simulink model "Stepper_Model_Statespace_Controller"  (R2017a)
settings: Solver=VariableStepAuto  StartTime=0.0  StopTime=15  FixedStep=0.01  RelTol=1e-3
undefined symbols (not defined in the file): Ad, Bd, Cd, Dd, Ptheta0, T, theta0
libraries: simulink x2
settings Model: Creator=Patrick  LastModifiedBy=Patrick

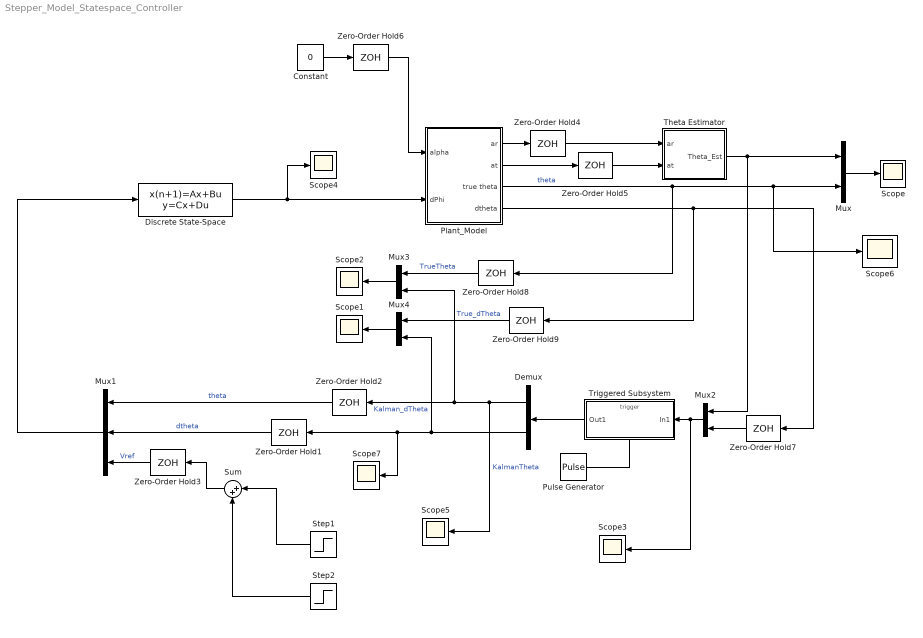
== system Stepper_Model_Statespace_Controller ==
  Constant : Constant  Value=0
  Demux : Demux  Outputs=2
  Discrete State-Space : DiscreteStateSpace  A=Ad  B=Bd  C=Cd  D=Dd  SampleTime=T
  Mux{,2..4} (4 alike) : Mux  Inputs=2
  Mux1 : Mux  Inputs=3
  Plant_Model : Subsystem
  Pulse Generator : DiscretePulseGenerator  PulseType=Time based  Period=T  PulseWidth=50
  Scope{,1..7} (8 alike) : Scope
  Step1 : Step  Time=5  After=.5  SampleTime=0
  Step2 : Step  Time=10  After=0  SampleTime=0
  Sum : Sum  Inputs=|++
  Theta Estimator : Subsystem
  Triggered Subsystem : Subsystem  TreatAsAtomicUnit=on
  Zero-Order Hold{1..9} (9 alike) : ZeroOrderHold  SampleTime=T
  wires:
  Mux/1 -> Scope/1
  Plant_Model/3(true theta) -> Scope6/1, Mux/2, Zero-Order Hold8/1  "theta"
  Mux1/1 -> Discrete State-Space/1
  Discrete State-Space/1 -> Scope4/1, Plant_Model/2(dPhi)
  Zero-Order Hold1/1 -> Mux1/2  "dtheta"
  Zero-Order Hold2/1 -> Mux1/1  "theta"
  Zero-Order Hold3/1 -> Mux1/3  "Vref"
  Plant_Model/1(ar) -> Zero-Order Hold4/1
  Zero-Order Hold4/1 -> Theta Estimator/1(ar)
  Zero-Order Hold5/1 -> Theta Estimator/2(at)
  Plant_Model/2(at) -> Zero-Order Hold5/1
  Theta Estimator/1(Theta_Est) -> Mux/1, Mux2/1
  Triggered Subsystem/1(Out1) -> Demux/1
  Mux2/1 -> Scope3/1, Triggered Subsystem/1(In1)
  Plant_Model/4(dtheta) -> Zero-Order Hold7/1, Zero-Order Hold9/1
  Mux3/1 -> Scope2/1
  Mux4/1 -> Scope1/1
  Demux/2 -> Scope7/1, Zero-Order Hold1/1, Mux4/2  "Kalman_dTheta"
  Demux/1 -> Scope5/1, Zero-Order Hold2/1, Mux3/2  "KalmanTheta"
  Pulse Generator/1 -> Triggered Subsystem/Trigger
  Zero-Order Hold7/1 -> Mux2/2
  Constant/1 -> Zero-Order Hold6/1
  Zero-Order Hold6/1 -> Plant_Model/1("alpha ")
  Zero-Order Hold8/1 -> Mux3/1  "TrueTheta"
  Zero-Order Hold9/1 -> Mux4/1  "True_dTheta"
  Sum/1 -> Zero-Order Hold3/1
  Step1/1 -> Sum/1
  Step2/1 -> Sum/2

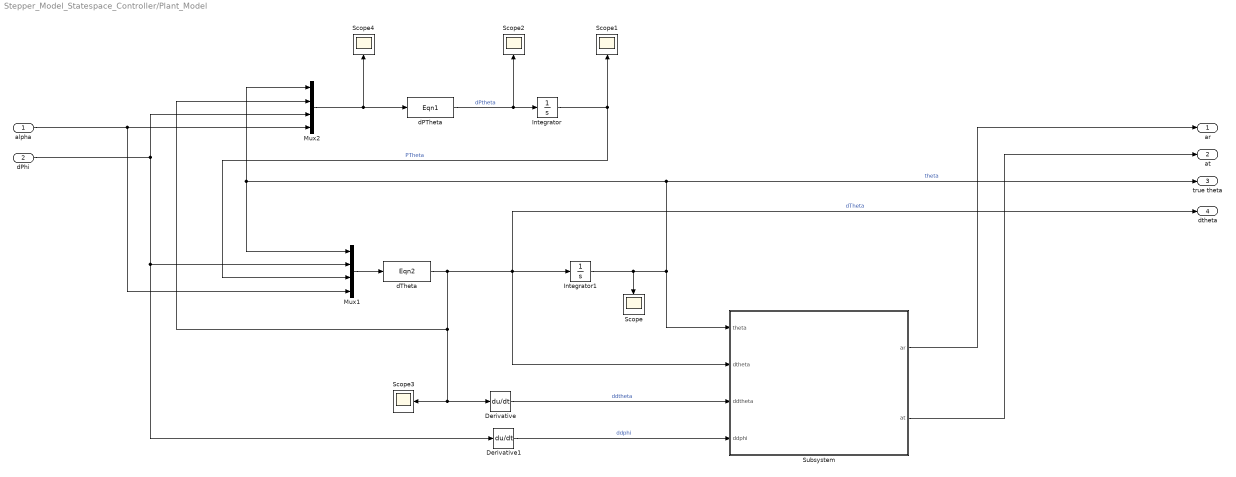
== system Stepper_Model_Statespace_Controller/Plant_Model ==
  "alpha " : Inport
  dPhi : Inport  Port=2
  Derivative : Derivative
  Derivative1 : Derivative
  Integrator : Integrator  InitialCondition=Ptheta0
  Integrator1 : Integrator  InitialCondition=theta0
  Mux1 : Mux  Inputs=[1 1 1 1]
  Mux2 : Mux  Inputs=[1 1 1 1]
  Scope{,1..4} (5 alike) : Scope
  Subsystem : Subsystem
  dPTheta : MATLABFcn  MATLABFcn=Eqn1  OutputDimensions=[1 1]  Output1D=off
  dTheta : MATLABFcn  MATLABFcn=Eqn2  OutputDimensions=[1 1]  Output1D=off
  ar : Outport  PortDimensions=[1 1]
  at : Outport  Port=2  PortDimensions=[1 1]
  true theta : Outport  Port=3  PortDimensions=[1 1]
  dtheta : Outport  Port=4  PortDimensions=[1 1]
  wires:
  Integrator/1 -> Mux1/3, Scope1/1  "PTheta"
  dPTheta/1 -> Integrator/1, Scope2/1  "dPtheta"
  dTheta/1 -> Subsystem/2(dtheta), dtheta/1, Integrator1/1, Scope3/1, Derivative/1, Mux2/2  "dTheta"
  Mux2/1 -> dPTheta/1, Scope4/1
  Mux1/1 -> dTheta/1
  Derivative/1 -> Subsystem/3(ddtheta)  "ddtheta"
  Derivative1/1 -> Subsystem/4(ddphi)  "ddphi"
  Integrator1/1 -> Subsystem/1(theta), Mux2/1, Mux1/1, true theta/1, Scope/1  "theta"
  Subsystem/2(at) -> at/1
  Subsystem/1(ar) -> ar/1
  dPhi/1 -> Derivative1/1, Mux1/2, Mux2/3
  "alpha "/1 -> Mux1/4, Mux2/4

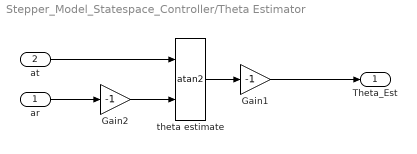
== system Stepper_Model_Statespace_Controller/Theta Estimator ==
  ar : Inport
  at : Inport  Port=2
  Gain1 : Gain  Gain=-1
  Gain2 : Gain  Gain=-1
  theta estimate : Trigonometry  Operator=atan2  OutputSignalType=real
  Theta_Est : Outport
  wires:
  ar/1 -> Gain2/1
  at/1 -> theta estimate/1
  Gain2/1 -> theta estimate/2
  theta estimate/1 -> Gain1/1
  Gain1/1 -> Theta_Est/1

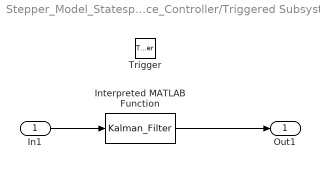
== system Stepper_Model_Statespace_Controller/Triggered Subsystem ==
  In1 : Inport
  Trigger : TriggerPort  VariantControl=Variant
  Interpreted MATLAB Function : MATLABFcn  MATLABFcn=Kalman_Filter  OutputDimensions=[2, 1]  Output1D=off
  Out1 : Outport
  wires:
  In1/1 -> Interpreted MATLAB Function/1
  Interpreted MATLAB Function/1 -> Out1/1

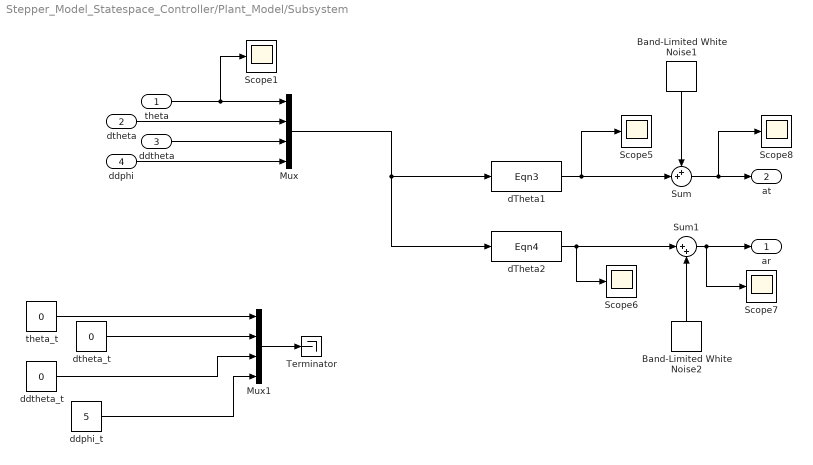
== system Stepper_Model_Statespace_Controller/Plant_Model/Subsystem ==
  theta : Inport
  dtheta : Inport  Port=2
  ddtheta : Inport  Port=3
  ddphi : Inport  Port=4
  Band-Limited White Noise1 : simulink/Sources/Band-Limited White Noise  Cov=[0.0000001]  Ts=.01  seed=[23341]
  Band-Limited White Noise2 : simulink/Sources/Band-Limited White Noise  Cov=[0.00000001]  Ts=.01  seed=[23341]
  Mux : Mux
  Mux1 : Mux
  Scope{1,5..8} (5 alike) : Scope
  Sum : Sum  Inputs=++|
  Sum1 : Sum  Inputs=|++
  Terminator : Terminator
  dTheta1 : MATLABFcn  MATLABFcn=Eqn3  OutputDimensions=[1 1]  Output1D=off
  dTheta2 : MATLABFcn  MATLABFcn=Eqn4  OutputDimensions=[1 1]  Output1D=off
  ddphi_t : Constant  Value=5
  ddtheta_t : Constant  Value=0
  dtheta_t : Constant  Value=0
  theta_t : Constant  Value=0
  ar : Outport  PortDimensions=[1 1]
  at : Outport  Port=2  PortDimensions=[1 1]
  wires:
  theta/1 -> Scope1/1, Mux/1
  dtheta/1 -> Mux/2
  Sum/1 -> at/1, Scope8/1
  dTheta2/1 -> Sum1/1, Scope6/1
  Sum1/1 -> ar/1, Scope7/1
  dTheta1/1 -> Sum/2, Scope5/1
  ddphi/1 -> Mux/4
  ddtheta/1 -> Mux/3
  Band-Limited White Noise1/1 -> Sum/1
  Band-Limited White Noise2/1 -> Sum1/2
  ddphi_t/1 -> Mux1/4
  theta_t/1 -> Mux1/1
  dtheta_t/1 -> Mux1/2
  ddtheta_t/1 -> Mux1/3
  Mux/1 -> dTheta1/1, dTheta2/1
  Mux1/1 -> Terminator/1
